simulink subsystem "UserInputsFocQepHost"  (R2024b)
settings: Solver=VariableStepAuto  StartTime=0.0  StopTime=10.0  RelTol=1e-3
libraries: simulink x3
settings Model: Creator=The MathWorks, Inc.  LastModifiedBy=I67977
settings RTWCC: GPUComputeCapability=3.5

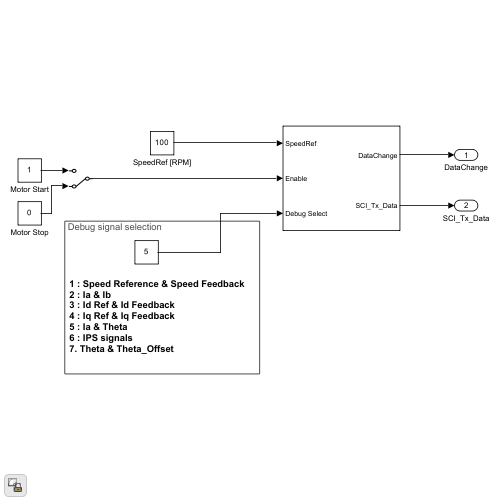
[thumbnail: Simulink's stored preview of the top-level diagram]
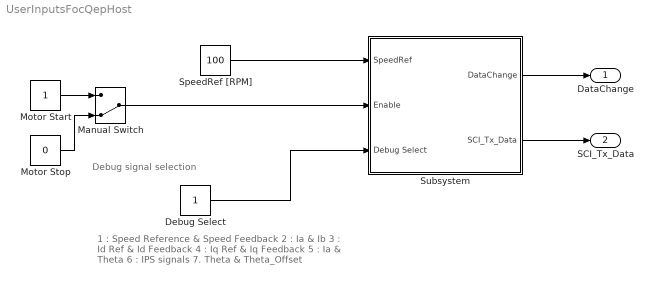
== system UserInputsFocQepHost ==
  note: Debug signal selection
  note: 1 : Speed Reference & Speed Feedback
      | 2 : Ia & Ib
      | 3 : Id Ref & Id Feedback
      | 4 : Iq Ref & Iq Feedback
      | 5 : Ia & Theta
      | 6 : IPS signals
      | 7. Theta & Theta_Offset
  Debug Select : Constant  OutDataTypeStr=uint8  SampleTime=-1
  Manual Switch : ManualSwitch  CurrentSetting=0
  Motor Start : Constant  OutDataTypeStr=uint16  SampleTime=-1
  Motor Stop : Constant  Value=0  OutDataTypeStr=uint16  SampleTime=-1
  SpeedRef [RPM] : Constant  Value=100  OutDataTypeStr=int16  SampleTime=-1
  Subsystem : Subsystem
  DataChange : Outport
  SCI_Tx_Data : Outport  Port=2
  wires:
  Subsystem/1(DataChange) -> DataChange/1
  Subsystem/2(SCI_Tx_Data) -> SCI_Tx_Data/1
  Motor Stop/1 -> Manual Switch/2
  Motor Start/1 -> Manual Switch/1
  Manual Switch/1 -> Subsystem/2(Enable)
  Debug Select/1 -> Subsystem/3(Debug Select)
  SpeedRef [RPM]/1 -> Subsystem/1(SpeedRef)

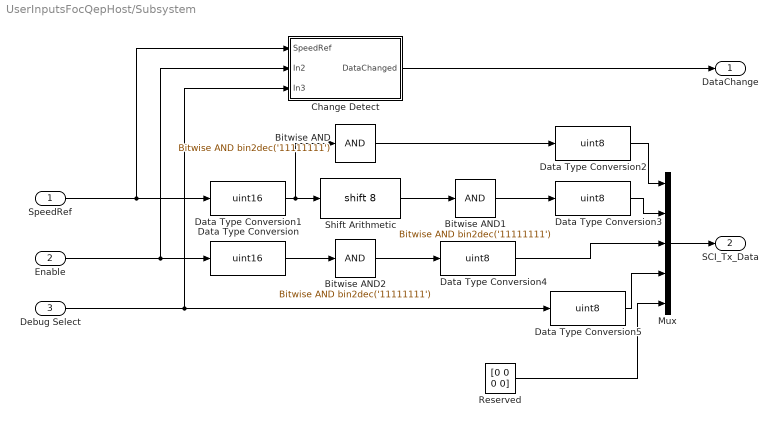
== system UserInputsFocQepHost/Subsystem ==
  SpeedRef : Inport
  Enable : Inport  Port=2
  Debug Select : Inport  Port=3
  Bitwise AND : simulink/Logic and Bit Operations/Bitwise Operator  logicop=AND  UseBitMask=on  BitMask=bin2dec('11111111')  BitMaskRealWorld=Stored Integer
  Bitwise AND1 : simulink/Logic and Bit Operations/Bitwise Operator  logicop=AND  UseBitMask=on  BitMask=bin2dec('11111111')  BitMaskRealWorld=Stored Integer
  Bitwise AND2 : simulink/Logic and Bit Operations/Bitwise Operator  logicop=AND  UseBitMask=on  BitMask=bin2dec('11111111')  BitMaskRealWorld=Stored Integer
  Change Detect : Subsystem
  Data Type Conversion : DataTypeConversion  OutDataTypeStr=uint16  ConvertRealWorld=Stored Integer (SI)  RndMeth=Simplest  SaturateOnIntegerOverflow=off
  Data Type Conversion1 : DataTypeConversion  OutDataTypeStr=uint16  ConvertRealWorld=Stored Integer (SI)  RndMeth=Simplest  SaturateOnIntegerOverflow=off
  Data Type Conversion{2..5} (4 alike) : DataTypeConversion  OutDataTypeStr=uint8  ConvertRealWorld=Stored Integer (SI)  RndMeth=Simplest  SaturateOnIntegerOverflow=off
  Mux : Mux  Inputs=5
  Reserved : Constant  Value=[0 0 0 0]  OutDataTypeStr=uint8  SampleTime=-1
  Shift Arithmetic : ArithShift  BitShiftNumber=8
  DataChange : Outport
  SCI_Tx_Data : Outport  Port=2
  wires:
  SpeedRef/1 -> Data Type Conversion1/1, Change Detect/1(SpeedRef)
  Change Detect/1(DataChanged) -> DataChange/1
  Mux/1 -> SCI_Tx_Data/1
  Enable/1 -> Data Type Conversion/1, Change Detect/2(In2)
  Data Type Conversion/1 -> Bitwise AND2/1
  Shift Arithmetic/1 -> Bitwise AND1/1
  Data Type Conversion1/1 -> Shift Arithmetic/1, Bitwise AND/1
  Bitwise AND2/1 -> Data Type Conversion4/1
  Bitwise AND/1 -> Data Type Conversion2/1
  Bitwise AND1/1 -> Data Type Conversion3/1
  Data Type Conversion4/1 -> Mux/3
  Debug Select/1 -> Data Type Conversion5/1, Change Detect/3(In3)
  Data Type Conversion2/1 -> Mux/1
  Data Type Conversion5/1 -> Mux/4
  Data Type Conversion3/1 -> Mux/2
  Reserved/1 -> Mux/5

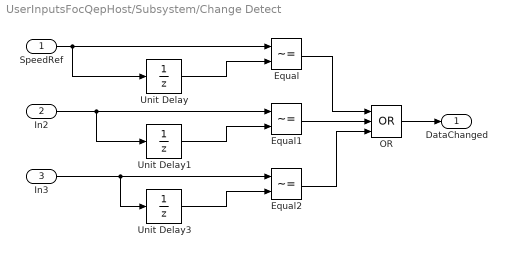
== system UserInputsFocQepHost/Subsystem/Change Detect ==
  SpeedRef : Inport
  In2 : Inport  Port=2
  In3 : Inport  Port=3
  Equal : RelationalOperator  Operator=~=  OutDataTypeStr=boolean  RndMeth=Simplest  InputSameDT=off
  Equal1 : RelationalOperator  Operator=~=  OutDataTypeStr=boolean  RndMeth=Simplest  InputSameDT=off
  Equal2 : RelationalOperator  Operator=~=  OutDataTypeStr=boolean  RndMeth=Simplest  InputSameDT=off
  OR : Logic  Operator=OR  Inputs=3  IconShape=distinctive  AllPortsSameDT=off  OutDataTypeStr=boolean
  Unit Delay : UnitDelay  SampleTime=-1  HasFrameUpgradeWarning=on
  Unit Delay1 : UnitDelay  SampleTime=-1  HasFrameUpgradeWarning=on
  Unit Delay3 : UnitDelay  SampleTime=-1  HasFrameUpgradeWarning=on
  DataChanged : Outport
  wires:
  Unit Delay3/1 -> Equal2/2
  Unit Delay1/1 -> Equal1/2
  SpeedRef/1 -> Equal/1, Unit Delay/1
  In2/1 -> Equal1/1, Unit Delay1/1
  Equal/1 -> OR/1
  Unit Delay/1 -> Equal/2
  Equal1/1 -> OR/2
  In3/1 -> Equal2/1, Unit Delay3/1
  OR/1 -> DataChanged/1
  Equal2/1 -> OR/3
